simulink model "MPO_braking_system"  (R2021b)
settings: Solver=VariableStepAuto  StartTime=0.0  StopTime=10  FixedStep=0.0001  MaxStep=0.01  RelTol=1e-3  EnableMultiTasking=on
PreLoadFcn:
  | sdl_braking_caliper_disk_brake_input
InitFcn:
  | f10 = 5; f11 = f10; f12 = f10;
  | f20 = 5; f21 = f20; f22 = f20;
undefined symbols (not defined in the file or in its folder): fcdb, tpc
libraries: fl_lib x154, nesl_utility x45, SimscapeFluids_lib x6, sdl_lib x4
(part 3 of 3)

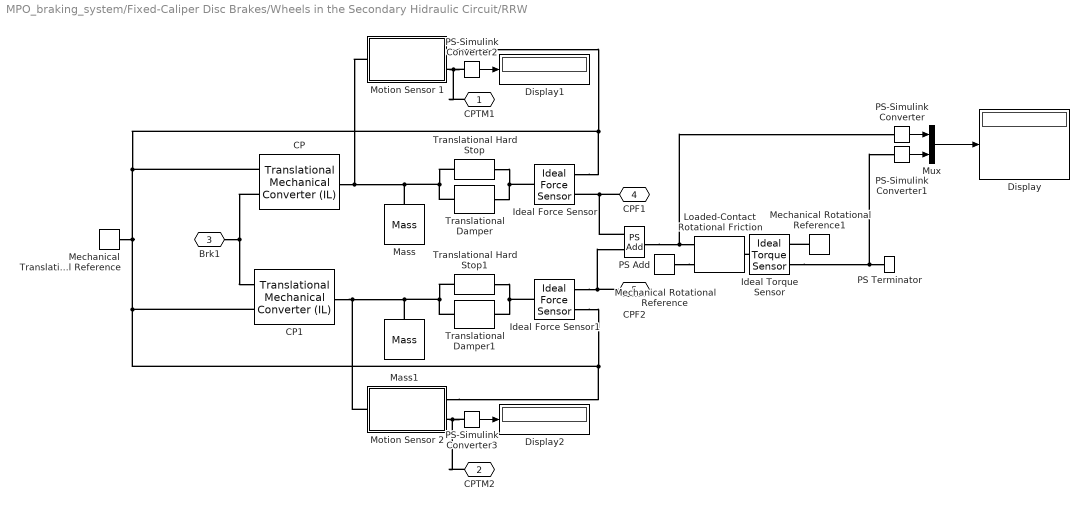
== system MPO_braking_system/Fixed-Caliper Disc Brakes/Wheels in the Secondary Hidraulic Circuit/RRW ==
  CP : fl_lib/Isothermal Liquid/Elements/Translational Mechanical Converter (IL)  mech_orientation=foundation.enum.MechOrientationTranslational.Positive  displacement_spec=foundation.enum.DisplacementSpec.Calculate  x0=0 m  interface_area=fcdb.area m^2  dead_volume=fcdb.deadV m^3  pressure_spec=foundation.enum.pressure_spec.atmospheric  environment_pressure=0.101325 MPa  dynamic_compressibility=simscape.enum.onoff.on  p0=tpc.pRes Pa
      settings: SourceProductBaseCode=SS  InternalSimscapePortConfiguration="{\"Bottom\":[],\"Left\":[{\"id\":\"A\",\"label\":\"A\",\"type\":\"foundation.isothermal_liquid.isothermal_liquid\"},{\"id\":\"C\",\"label\":\"C\",\"type\":\"foundation.mechanical.translational.translational\"}],\"Right\":[{\"id\":\"R\",\"label\":\"R\",\"type\":\"foundation.mechanical.translational.translational\"}],\"Top\":[]}"
  CP1 : fl_lib/Isothermal Liquid/Elements/Translational Mechanical Converter (IL)  mech_orientation=foundation.enum.MechOrientationTranslational.Positive  displacement_spec=foundation.enum.DisplacementSpec.Calculate  x0=0 m  interface_area=fcdb.area m^2  dead_volume=fcdb.deadV m^3  pressure_spec=foundation.enum.pressure_spec.atmospheric  environment_pressure=0.101325 MPa  dynamic_compressibility=simscape.enum.onoff.on  p0=tpc.pRes Pa
      settings: SourceProductBaseCode=SS  InternalSimscapePortConfiguration="{\"Bottom\":[],\"Left\":[{\"id\":\"A\",\"label\":\"A\",\"type\":\"foundation.isothermal_liquid.isothermal_liquid\"},{\"id\":\"C\",\"label\":\"C\",\"type\":\"foundation.mechanical.translational.translational\"}],\"Right\":[{\"id\":\"R\",\"label\":\"R\",\"type\":\"foundation.mechanical.translational.translational\"}],\"Top\":[]}"
  Display : Display
  Display1 : Display
  Display2 : Display
  Ideal Force Sensor : fl_lib/Mechanical/Mechanical Sensors/Ideal Force Sensor
  Ideal Force Sensor1 : fl_lib/Mechanical/Mechanical Sensors/Ideal Force Sensor
  Ideal Torque Sensor : fl_lib/Mechanical/Mechanical Sensors/Ideal Torque Sensor
  Loaded-Contact Rotational Friction : sdl_lib/Brakes & Detents/Rotational/Loaded-Contact Rotational Friction  geometry_model=sdl.enum.friction_geometry.radius  r_eff=fcdb.reff m  d_o=150 mm  d_i=100 mm  friction_model=sdl.enum.friction_model_TLU_thermal.fixed  mu_w_vector=[0, 100, 1000] rad/s  temperature_TLU=[280, 300, 320] K  mu_static=fcdb.statFric  mu_static_vector=[.4, .38, .36]  mu_coulomb=fcdb.kinFric  mu_coulomb_vector=[.3, .22, .19]  mu_coulomb_temp_vector=[.3, .28, .25]  mu_coulomb_matrix=[.34, .32, .3; .3, .28, .25; .25, .2, .15]  mu_interp_method=simscape.enum.interpolation.linear  mu_extrap_method=simscape.enum.extrapolation.linear  w_tol=0.001 rad/s  force_min=1 N  mu_visc=fcdb.dampDisk N*m/(rad/s)  initial_state_locked=sdl.enum.initial_lock.locked  enable_faults=simscape.enum.onoff.off  fault_type=sdl.enum.clutchFault.lock  external_fault=simscape.enum.onoff.off  temporal_fault=simscape.enum.onoff.off  fault_time=5 s  report_fault=simscape.enum.assert.action.none  thermal_mass=50 kJ/K  T_init=300 K
      settings: SourceProductBaseCode=LD  InternalSimscapePortConfiguration="{\"Bottom\":[],\"Left\":[{\"id\":\"N\",\"label\":\"N\",\"type\":\"input\"},{\"id\":\"B\",\"label\":\"B\",\"type\":\"foundation.mechanical.rotational.rotational\"}],\"Right\":[{\"id\":\"F\",\"label\":\"F\",\"type\":\"foundation.mechanical.rotational.rotational\"}],\"Top\":[]}"
  Mass : fl_lib/Mechanical/Translational Elements/Mass  mass=fcdb.mass kg  num_ports=foundation.enum.numPorts2.one  v_specify=off  v_priority=High  v=0 m/s  v_nominal_specify=off  v_nominal_unit=m/s  v_nominal_value=1  f_specify=off  f_priority=None  f=0 N  f_nominal_specify=off  f_nominal_unit=N  f_nominal_value=1
  Mass1 : fl_lib/Mechanical/Translational Elements/Mass  mass=fcdb.mass kg  num_ports=foundation.enum.numPorts2.one  v_specify=off  v_priority=High  v=0 m/s  v_nominal_specify=off  v_nominal_unit=m/s  v_nominal_value=1  f_specify=off  f_priority=None  f=0 N  f_nominal_specify=off  f_nominal_unit=N  f_nominal_value=1
  Mechanical Rotational Reference : fl_lib/Mechanical/Rotational Elements/Mechanical Rotational Reference
  Mechanical Rotational Reference1 : fl_lib/Mechanical/Rotational Elements/Mechanical Rotational Reference
  Mechanical Translational Reference : fl_lib/Mechanical/Translational Elements/Mechanical Translational Reference
  Motion Sensor 1 : Subsystem
  Motion Sensor 2 : Subsystem
  Mux : Mux  Inputs=2
  PS Add : fl_lib/Physical Signals/Functions/PS Add
  PS Terminator : fl_lib/Physical Signals/Sinks/PS Terminator
  PS-Simulink Converter{,1..3} (4 alike) : nesl_utility/PS-Simulink Converter  PhysicalDomain=network_engine_domain  SubClassName=ps_output  LeftPortType=input  RightPortType=output  PseudoPeriodic=off  Frequencies=[]  Unit=inherit  AffineConversion=off
      settings: SourceProductBaseCode=PW,SS
  Translational Damper : fl_lib/Mechanical/Translational Elements/Translational Damper  D=fcdb.damp N/(m/s)  v_specify=off  v_priority=None  v=0 m/s  v_nominal_specify=off  v_nominal_unit=m/s  v_nominal_value=1  f_specify=off  f_priority=None  f=0 N  f_nominal_specify=off  f_nominal_unit=N  f_nominal_value=1
  Translational Damper1 : fl_lib/Mechanical/Translational Elements/Translational Damper  D=fcdb.damp N/(m/s)  v_specify=off  v_priority=None  v=0 m/s  v_nominal_specify=off  v_nominal_unit=m/s  v_nominal_value=1  f_specify=off  f_priority=None  f=0 N  f_nominal_specify=off  f_nominal_unit=N  f_nominal_value=1
  Translational Hard Stop : fl_lib/Mechanical/Translational Elements/Translational Hard Stop  upper_bnd=fcdb.runClear m  lower_bnd=0 m  stiff_up=fcdb.complianceF N/m  stiff_low=fcdb.hss N/m  D_up=fcdb.damp N/(m/s)  D_low=fcdb.hsd N/(m/s)  model=simscape.enum.hardstop.smooth  transition=0.1 mm  v_specify=off  v_priority=None  v=0 m/s  v_nominal_specify=off  v_nominal_unit=m/s  v_nominal_value=1  f_specify=off  f_priority=None  f=0 N  f_nominal_specify=off  f_nominal_unit=N  f_nominal_value=1  x_specify=off  x_priority=High  x=0 m  x_nominal_specify=off  x_nominal_unit=m  x_nominal_value=1
  Translational Hard Stop1 : fl_lib/Mechanical/Translational Elements/Translational Hard Stop  upper_bnd=fcdb.runClear m  lower_bnd=0 m  stiff_up=fcdb.complianceF N/m  stiff_low=fcdb.hss N/m  D_up=fcdb.damp N/(m/s)  D_low=fcdb.hsd N/(m/s)  model=simscape.enum.hardstop.smooth  transition=0.1 mm  v_specify=off  v_priority=None  v=0 m/s  v_nominal_specify=off  v_nominal_unit=m/s  v_nominal_value=1  f_specify=off  f_priority=None  f=0 N  f_nominal_specify=off  f_nominal_unit=N  f_nominal_value=1  x_specify=off  x_priority=High  x=0 m  x_nominal_specify=off  x_nominal_unit=m  x_nominal_value=1
  CPTM1 : PMIOPort  Side=Right
  CPTM2 : PMIOPort  Port=2  Side=Right
  Brk1 : PMIOPort  Port=3  Side=Left
  CPF1 : PMIOPort  Port=4  Side=Right
  CPF2 : PMIOPort  Port=5  Side=Right
  wires:
  PS-Simulink Converter/1 -> Mux/1
  PS-Simulink Converter1/1 -> Mux/2
  Mux/1 -> Display/1
  PS-Simulink Converter2/1 -> Display1/1
  PS-Simulink Converter3/1 -> Display2/1
  connections:
  Translational Hard Stop/LConn1 -- Translational Damper/LConn1 -- Mass/LConn1 -- Motion Sensor 1/LConn1 -- CP/RConn1
  Ideal Force Sensor/LConn1 -- Translational Hard Stop/RConn1 -- Translational Damper/RConn1
  Mechanical Translational Reference/LConn1 -- Ideal Force Sensor/RConn1 -- Motion Sensor 1/RConn1 -- CP/LConn2 -- CP1/LConn2 -- Ideal Force Sensor1/RConn1 -- Motion Sensor 2/RConn1
  Mechanical Rotational Reference/LConn1 -- Loaded-Contact Rotational Friction/LConn2
  Ideal Torque Sensor/LConn1 -- Loaded-Contact Rotational Friction/RConn1
  Mass1/LConn1 -- Translational Hard Stop1/LConn1 -- Translational Damper1/LConn1 -- CP1/RConn1 -- Motion Sensor 2/LConn1
  Translational Damper1/RConn1 -- Translational Hard Stop1/RConn1 -- Ideal Force Sensor1/LConn1
  CPF1/RConn1 -- PS Add/LConn1 -- Ideal Force Sensor/RConn2
  CPF2/RConn1 -- Ideal Force Sensor1/RConn2 -- PS Add/LConn2
  PS Add/RConn1 -- PS-Simulink Converter/LConn1 -- Loaded-Contact Rotational Friction/LConn1
  Mechanical Rotational Reference1/LConn1 -- Ideal Torque Sensor/RConn1
  Ideal Torque Sensor/RConn2 -- PS-Simulink Converter1/LConn1 -- PS Terminator/LConn1
  Brk1/RConn1 -- CP/LConn1 -- CP1/LConn1
  Motion Sensor 1/RConn2 -- PS-Simulink Converter2/LConn1 -- CPTM1/RConn1
  Motion Sensor 2/RConn2 -- PS-Simulink Converter3/LConn1 -- CPTM2/RConn1

== system MPO_braking_system/Fixed-Caliper Disc Brakes/Wheels in the Secondary Hidraulic Circuit/Subsystem2 ==
  PS Add : fl_lib/Physical Signals/Functions/PS Add
  PS Constant : fl_lib/Physical Signals/Sources/PS Constant  constant=2 m
  PS Divide : fl_lib/Physical Signals/Functions/PS Divide
      settings: SourceProductBaseCode=SS
  Conn1 : PMIOPort  Side=Left
  Conn2 : PMIOPort  Port=2  Side=Right
  Conn3 : PMIOPort  Port=3  Side=Left
  connections:
  PS Constant/RConn1 -- PS Divide/LConn2
  PS Divide/LConn1 -- PS Add/RConn1
  Conn3/RConn1 -- PS Add/LConn2
  PS Divide/RConn1 -- Conn2/RConn1
  PS Add/LConn1 -- Conn1/RConn1

== system MPO_braking_system/Fixed-Caliper Disc Brakes/Wheels in the Secondary Hidraulic Circuit/Subsystem3 ==
  PS Add : fl_lib/Physical Signals/Functions/PS Add
  PS Constant : fl_lib/Physical Signals/Sources/PS Constant  constant=2 m
  PS Divide : fl_lib/Physical Signals/Functions/PS Divide
      settings: SourceProductBaseCode=SS
  Conn1 : PMIOPort  Side=Left
  Conn2 : PMIOPort  Port=2  Side=Right
  Conn3 : PMIOPort  Port=3  Side=Left
  connections:
  PS Constant/RConn1 -- PS Divide/LConn2
  PS Divide/LConn1 -- PS Add/RConn1
  Conn3/RConn1 -- PS Add/LConn2
  PS Divide/RConn1 -- Conn2/RConn1
  PS Add/LConn1 -- Conn1/RConn1

== system MPO_braking_system/Fixed-Caliper Disc Brakes/Wheels in the Secondary Hidraulic Circuit/Subsystem6 ==
  PS Add : fl_lib/Physical Signals/Functions/PS Add
  PS Constant : fl_lib/Physical Signals/Sources/PS Constant  constant=2 N
  PS Divide : fl_lib/Physical Signals/Functions/PS Divide
      settings: SourceProductBaseCode=SS
  Conn1 : PMIOPort  Side=Left
  Conn2 : PMIOPort  Port=2  Side=Right
  Conn3 : PMIOPort  Port=3  Side=Left
  connections:
  PS Constant/RConn1 -- PS Divide/LConn2
  PS Divide/LConn1 -- PS Add/RConn1
  Conn3/RConn1 -- PS Add/LConn2
  PS Divide/RConn1 -- Conn2/RConn1
  PS Add/LConn1 -- Conn1/RConn1

== system MPO_braking_system/Fixed-Caliper Disc Brakes/Wheels in the Secondary Hidraulic Circuit/Subsystem7 ==
  PS Add : fl_lib/Physical Signals/Functions/PS Add
  PS Constant : fl_lib/Physical Signals/Sources/PS Constant  constant=2 N
  PS Divide : fl_lib/Physical Signals/Functions/PS Divide
      settings: SourceProductBaseCode=SS
  Conn1 : PMIOPort  Side=Left
  Conn2 : PMIOPort  Port=2  Side=Right
  Conn3 : PMIOPort  Port=3  Side=Left
  connections:
  PS Constant/RConn1 -- PS Divide/LConn2
  PS Divide/LConn1 -- PS Add/RConn1
  Conn3/RConn1 -- PS Add/LConn2
  PS Divide/RConn1 -- Conn2/RConn1
  PS Add/LConn1 -- Conn1/RConn1

== system MPO_braking_system/Fixed-Caliper Disc Brakes/Wheels in the Primary Hidraulic Circuit/FLW/Motion Sensor 1 ==
  Ideal Translational Motion Sensor : fl_lib/Mechanical/Mechanical Sensors/Ideal Translational Motion Sensor  offset=0 m
  PS Terminator1 : fl_lib/Physical Signals/Sinks/PS Terminator
  C : PMIOPort  Side=Right
  P : PMIOPort  Port=2  Side=Right
  R : PMIOPort  Port=3  Side=Left
  connections:
  PS Terminator1/LConn1 -- Ideal Translational Motion Sensor/RConn2
  Ideal Translational Motion Sensor/LConn1 -- R/RConn1
  Ideal Translational Motion Sensor/RConn3 -- P/RConn1
  Ideal Translational Motion Sensor/RConn1 -- C/RConn1

== system MPO_braking_system/Fixed-Caliper Disc Brakes/Wheels in the Primary Hidraulic Circuit/FLW/Motion Sensor 2 ==
  Ideal Translational Motion Sensor : fl_lib/Mechanical/Mechanical Sensors/Ideal Translational Motion Sensor  offset=0 m
  PS Terminator1 : fl_lib/Physical Signals/Sinks/PS Terminator
  C : PMIOPort  Side=Right
  P : PMIOPort  Port=2  Side=Right
  R : PMIOPort  Port=3  Side=Left
  connections:
  PS Terminator1/LConn1 -- Ideal Translational Motion Sensor/RConn2
  Ideal Translational Motion Sensor/LConn1 -- R/RConn1
  Ideal Translational Motion Sensor/RConn3 -- P/RConn1
  Ideal Translational Motion Sensor/RConn1 -- C/RConn1

== system MPO_braking_system/Fixed-Caliper Disc Brakes/Wheels in the Primary Hidraulic Circuit/FRW/Motion Sensor 1 ==
  Ideal Translational Motion Sensor : fl_lib/Mechanical/Mechanical Sensors/Ideal Translational Motion Sensor  offset=0 m
  PS Terminator1 : fl_lib/Physical Signals/Sinks/PS Terminator
  C : PMIOPort  Side=Right
  P : PMIOPort  Port=2  Side=Right
  R : PMIOPort  Port=3  Side=Left
  connections:
  PS Terminator1/LConn1 -- Ideal Translational Motion Sensor/RConn2
  Ideal Translational Motion Sensor/LConn1 -- R/RConn1
  Ideal Translational Motion Sensor/RConn3 -- P/RConn1
  Ideal Translational Motion Sensor/RConn1 -- C/RConn1

== system MPO_braking_system/Fixed-Caliper Disc Brakes/Wheels in the Primary Hidraulic Circuit/FRW/Motion Sensor 2 ==
  Ideal Translational Motion Sensor : fl_lib/Mechanical/Mechanical Sensors/Ideal Translational Motion Sensor  offset=0 m
  PS Terminator1 : fl_lib/Physical Signals/Sinks/PS Terminator
  C : PMIOPort  Side=Right
  P : PMIOPort  Port=2  Side=Right
  R : PMIOPort  Port=3  Side=Left
  connections:
  PS Terminator1/LConn1 -- Ideal Translational Motion Sensor/RConn2
  Ideal Translational Motion Sensor/LConn1 -- R/RConn1
  Ideal Translational Motion Sensor/RConn3 -- P/RConn1
  Ideal Translational Motion Sensor/RConn1 -- C/RConn1

== system MPO_braking_system/Fixed-Caliper Disc Brakes/Wheels in the Secondary Hidraulic Circuit/RLW/Motion Sensor 1 ==
  Ideal Translational Motion Sensor : fl_lib/Mechanical/Mechanical Sensors/Ideal Translational Motion Sensor  offset=0 m
  PS Terminator1 : fl_lib/Physical Signals/Sinks/PS Terminator
  C : PMIOPort  Side=Right
  P : PMIOPort  Port=2  Side=Right
  R : PMIOPort  Port=3  Side=Left
  connections:
  PS Terminator1/LConn1 -- Ideal Translational Motion Sensor/RConn2
  Ideal Translational Motion Sensor/LConn1 -- R/RConn1
  Ideal Translational Motion Sensor/RConn3 -- P/RConn1
  Ideal Translational Motion Sensor/RConn1 -- C/RConn1

== system MPO_braking_system/Fixed-Caliper Disc Brakes/Wheels in the Secondary Hidraulic Circuit/RLW/Motion Sensor 2 ==
  Ideal Translational Motion Sensor : fl_lib/Mechanical/Mechanical Sensors/Ideal Translational Motion Sensor  offset=0 m
  PS Terminator1 : fl_lib/Physical Signals/Sinks/PS Terminator
  C : PMIOPort  Side=Right
  P : PMIOPort  Port=2  Side=Right
  R : PMIOPort  Port=3  Side=Left
  connections:
  PS Terminator1/LConn1 -- Ideal Translational Motion Sensor/RConn2
  Ideal Translational Motion Sensor/LConn1 -- R/RConn1
  Ideal Translational Motion Sensor/RConn3 -- P/RConn1
  Ideal Translational Motion Sensor/RConn1 -- C/RConn1

== system MPO_braking_system/Fixed-Caliper Disc Brakes/Wheels in the Secondary Hidraulic Circuit/RRW/Motion Sensor 1 ==
  Ideal Translational Motion Sensor : fl_lib/Mechanical/Mechanical Sensors/Ideal Translational Motion Sensor  offset=0 m
  PS Terminator1 : fl_lib/Physical Signals/Sinks/PS Terminator
  C : PMIOPort  Side=Right
  P : PMIOPort  Port=2  Side=Right
  R : PMIOPort  Port=3  Side=Left
  connections:
  PS Terminator1/LConn1 -- Ideal Translational Motion Sensor/RConn2
  Ideal Translational Motion Sensor/LConn1 -- R/RConn1
  Ideal Translational Motion Sensor/RConn3 -- P/RConn1
  Ideal Translational Motion Sensor/RConn1 -- C/RConn1

== system MPO_braking_system/Fixed-Caliper Disc Brakes/Wheels in the Secondary Hidraulic Circuit/RRW/Motion Sensor 2 ==
  Ideal Translational Motion Sensor : fl_lib/Mechanical/Mechanical Sensors/Ideal Translational Motion Sensor  offset=0 m
  PS Terminator1 : fl_lib/Physical Signals/Sinks/PS Terminator
  C : PMIOPort  Side=Right
  P : PMIOPort  Port=2  Side=Right
  R : PMIOPort  Port=3  Side=Left
  connections:
  PS Terminator1/LConn1 -- Ideal Translational Motion Sensor/RConn2
  Ideal Translational Motion Sensor/LConn1 -- R/RConn1
  Ideal Translational Motion Sensor/RConn3 -- P/RConn1
  Ideal Translational Motion Sensor/RConn1 -- C/RConn1

== matlab function MPO_braking_system/Push Rod Force Generator/Force Generation ==
  data: stop output; clock input; signal output; rate input
function [stop, signal] = fcn(clock, rate)


% linear signal
min_signal = 0;
max_signal = 4000;
signal = min(min_signal + rate*clock,max_signal);

if (signal == max_signal)
    stop = 1;
else
    stop = 0;
end

== stateflow chart MPO_braking_system/Hydraulic System 1/mpo1 ==
  state mpo_x1
    en:
    S1=[1,-1,-1,-1];
  state mpo_x2_1
    en:
    S1=[2,-1,-1,-1];
  state mpo_x2
    en:
    S1=[9,-1,-1,-1];
  state m_x3
    en:
    S1=[11,1,-1,-1];
  state m_x5
    en:
    S1=[8,-1,-1,1];
  state m_x4
    en:
    S1=[8,-1,1,-1];
  (default) -> mpo_x1
  mpo_x1 -> mpo_x2_1 : [F>500]
  mpo_x2_1 -> mpo_x2 : [P1<1.16e3*F-2.28e5-2e5]
  mpo_x2 -> m_x5 [order 1] : [Q12>1.18e-9*DF+1.5e-5]
  mpo_x2 -> m_x4 [order 2] : [Q11>1.18e-9*DF+1.5e-5 ]
  mpo_x2 -> m_x3 [order 3] : [Q11<1.18e-9*DF-1.5e-5]
  data: F input; DF input; P1 input; Q11 input; S1 output; Q12 input

== stateflow chart MPO_braking_system/Hydraulic System 2/mpo2 ==
  state mpo_x1
    en:
    S2=[1,-1,-1,-1];
  state mpo_x2_1
    en:
    S2=[2,-1,-1,-1];
  state mpo_x2
    en:
    S2=[9,-1,-1,-1];
  state m_x3
    en:
    S2=[11,1,-1,-1];
  state m_x5
    en:
    S2=[8,-1,-1,1];
  state m_x4
    en:
    S2=[8,-1,1,-1];
  (default) -> mpo_x1
  mpo_x1 -> mpo_x2_1 : [F>500]
  mpo_x2_1 -> mpo_x2 : [P1<1.16e3*F-2.28e5-2e5]
  mpo_x2 -> m_x5 [order 1] : [Q12>1.18e-9*DF+1.5e-5]
  mpo_x2 -> m_x4 [order 2] : [Q11>1.18e-9*DF+1.5e-5 ]
  mpo_x2 -> m_x3 [order 3] : [Q11<1.18e-9*DF-1.5e-5]
  data: F input; DF input; P1 input; Q11 input; S2 output; Q12 input
